simulink model "sys_ident1"  (R2020b)
settings: Solver=ode1  StartTime=0.0  StopTime=100  FixedStep=0.001  MaxStep=Ts  RelTol=1e-3
settings Model: Creator=sl  LastModifiedBy=a4327481
settings DataIOCC: SaveOutput=off  SaveTime=off
settings OptimizationCC: DefaultParameterBehavior=Inlined  EnhancedBackFolding=on  PassReuseOutputArgsAs=Individual arguments  ZeroExternalMemoryAtStartup=off  ZeroInternalMemoryAtStartup=off  OptimizeBlockOrder=speed  DifferentSizesBufferReuse=on  OptimizationCustomize=off  EfficientTunableParamExpr=on
settings DebuggingCC: InheritedTsInSrcMsg=none  ParameterPrecisionLossMsg=none  ParameterTunabilityLossMsg=error  UnconnectedInputMsg=none  UnconnectedOutputMsg=none  UnconnectedLineMsg=none
settings HardwareCC: ProdBitPerPointer=32  ProdBitPerSizeT=32  ProdBitPerPtrDiffT=32  ProdLargestAtomicInteger=Long  ProdLargestAtomicFloat=Double  ProdWordSize=32  ProdHWDeviceType=ARM Compatible->ARM Cortex
settings ModelReferenceCC: ParallelModelReferenceMATLABWorkerInit=Copy Base Workspace  ModelReferenceNumInstancesAllowed=Single
settings SFSimCC: MATLABDynamicMemAlloc=off
settings RTWCC: Description=Embedded Coder  SystemTargetFile=ert.tlc  GenCodeOnly=on  PackageGeneratedCodeAndArtifacts=on  TemplateMakefile=ert_default_tmf  GenerateReport=on  IncludeHyperlinkInReport=on  LaunchReport=on  GenerateTraceInfo=on  GenerateTraceReport=on  GenerateTraceReportSl=on  GenerateTraceReportSf=on  GenerateTraceReportEml=on
settings CodeAppCC: ForceParamTrailComments=on  IgnoreCustomStorageClasses=off  MaxIdLength=48  OperatorAnnotations=on  SimulinkDataObjDesc=on  SFDataObjDesc=on  MATLABFcnDesc=on  InsertBlockDesc=on  MATLABSourceComments=on
settings ERTTargetCC: TargetLangStandard=C99 (ISO)  GenerateSampleERTMain=on  LogVarNameModifier=none  SupportVariableSizeSignals=on  InlinedParameterPlacement=NonHierarchical  ERTCustomFileTemplate=example_file_process.tlc  ERTFilePackagingFormat=Compact

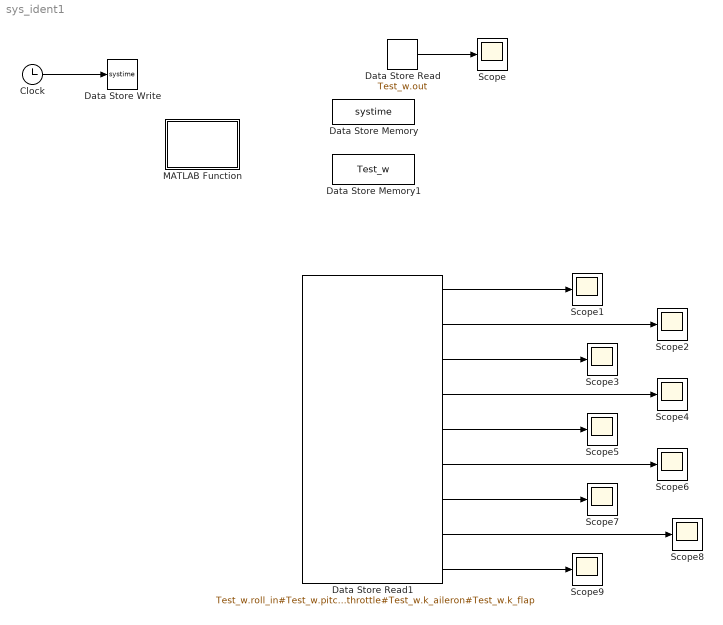
== system sys_ident1 ==
  Clock : Clock
  Data Store Memory : DataStoreMemory  DataStoreName=systime  ReadBeforeWriteMsg=warning  WriteAfterWriteMsg=warning  WriteAfterReadMsg=warning  InitialValue=systime  ShowAdditionalParam=off  OutDataTypeStr=double
  Data Store Memory1 : DataStoreMemory  DataStoreName=Test_w  ReadBeforeWriteMsg=warning  WriteAfterWriteMsg=warning  WriteAfterReadMsg=warning  InitialValue=Test_w  ShowAdditionalParam=off  OutDataTypeStr=Bus: Bus_Test_w
  Data Store Read : DataStoreRead  DataStoreName=Test_w  DataStoreElements=Test_w.out
  Data Store Read1 : DataStoreRead  DataStoreName=Test_w  DataStoreElements=Test_w.roll_in#Test_w.pitch_in#Test_w.yaw_in#Test_w.throttle_in#Test_w.k_rudder#Test_w.k_elevator#Test_w.k_throttle#Test_w.k_aileron#Test_w.k_flap
  Data Store Write : DataStoreWrite  DataStoreName=systime
  MATLAB Function : MATLAB Function  TreatAsAtomicUnit=on
  Scope{,1..9} (10 alike) : Scope
  wires:
  Clock/1 -> Data Store Write/1
  Data Store Read/1 -> Scope/1
  Data Store Read1/1 -> Scope1/1
  Data Store Read1/9 -> Scope9/1
  Data Store Read1/3 -> Scope3/1
  Data Store Read1/5 -> Scope5/1
  Data Store Read1/7 -> Scope7/1
  Data Store Read1/2 -> Scope2/1
  Data Store Read1/4 -> Scope4/1
  Data Store Read1/6 -> Scope6/1
  Data Store Read1/8 -> Scope8/1

== matlab function sys_ident1/MATLAB Function ==
  data: systime data_store_memory; Test_w data_store_memory
function fun()
global Test_w
        switch Test_w.mode
            case ENUM_Test_mode.step_w
                step_w();
            case ENUM_Test_mode.sin_w
                sin_w();
        end
    Test_w.roll_in=(Test_w.channel==ENUM_Test_channel.roll_in)*Test_w.out;
    Test_w.pitch_in=(Test_w.channel==ENUM_Test_channel.pitch_in)*Test_w.out;
    Test_w.yaw_in=(Test_w.channel==ENUM_Test_channel.yaw_in)*Test_w.out;
    Test_w.throttle_in=(Test_w.channel==ENUM_Test_channel.throttle_in)*Test_w.out;
    Test_w.k_rudder=(Test_w.channel==ENUM_Test_channel.k_rudder)*Test_w.out;
    Test_w.k_elevator=(Test_w.channel==ENUM_Test_channel.k_elevator)*Test_w.out;
    Test_w.k_throttle=(Test_w.channel==ENUM_Test_channel.k_throttle)*Test_w.out;
    Test_w.k_aileron=(Test_w.channel==ENUM_Test_channel.k_aileron)*Test_w.out;
    Test_w.k_flap=(Test_w.channel==ENUM_Test_channel.k_flap)*Test_w.out;   
end
